simulink model "simulacao_aeropendulo_LGR"  (R2021a)
settings: Solver=ode4  StartTime=0.0  StopTime=10  FixedStep=1e-3  RelTol=1e-3
values from neighbouring files (symbols this model uses):
  b = 0.006856    [aeropendulo_vars.m]
  g = 9.81    [aeropendulo_vars.m]
  I = 0.0264    [aeropendulo_vars.m]
  kh = 2.12829e-5    (= 2.12829e-05)    [aeropendulo_vars.m]
  Lh = 0.32    [aeropendulo_vars.m]
  m = 0.3182    [aeropendulo_vars.m]
  omega_barra = sqrt(m*g*sin(theta_barra)/(kh))    [aeropendulo_vars.m]
  theta_barra = theta_deg*pi/180    (= 1.3962634016)    [aeropendulo_vars.m]
libraries: aerolibconvert2 x1
settings Model: Creator=Luis Costa  LastModifiedBy=Luis Costa

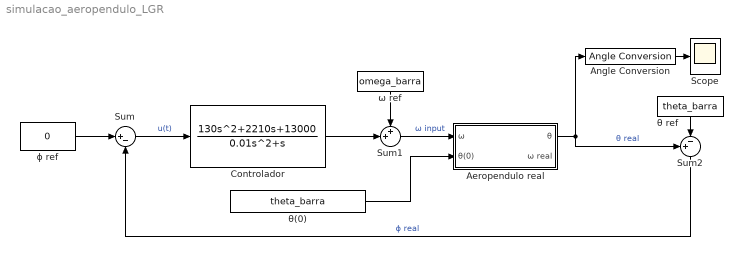
== system simulacao_aeropendulo_LGR ==
  Aeropendulo real : Subsystem
  Angle Conversion : aerolibconvert2/Angle Conversion  IU=rad  OU=deg
  Controlador : TransferFcn  Numerator=[130 2210 13000]  Denominator=[0.01 1 0]
  Scope : Scope
  Sum : Sum  Inputs=|+-
  Sum1 : Sum  Inputs=++|
  Sum2 : Sum  Inputs=+-|
  θ ref : Constant  Value=theta_barra
  θ(0) : Constant  Value=theta_barra
  ω ref : Constant  Value=omega_barra
  ϕ ref : Constant  Value=0
  wires:
  ω ref/1 -> Sum1/1
  θ ref/1 -> Sum2/2
  Sum1/1 -> Aeropendulo real/1(ω)  "ω input"
  Sum2/1 -> Sum/2  "ϕ real"
  Aeropendulo real/1(θ) -> Sum2/1, Angle Conversion/1  "θ real"
  Angle Conversion/1 -> Scope/1
  Sum/1 -> Controlador/1  "u(t)"
  θ(0)/1 -> Aeropendulo real/2(θ(0))
  ϕ ref/1 -> Sum/1
  Controlador/1 -> Sum1/2

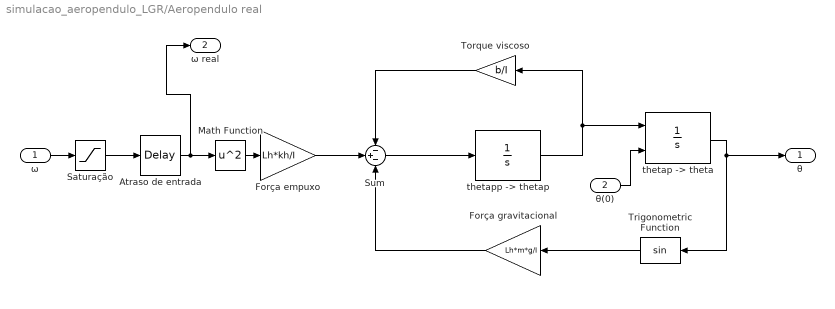
== system simulacao_aeropendulo_LGR/Aeropendulo real ==
  ω : Inport
  θ(0) : Inport  Port=2
  Atraso de entrada : TransportDelay  DelayTime=5e-3
  Força empuxo : Gain  Gain=Lh*kh/I  OutMin=[0]  OutMax=[375]
  Força gravitacional : Gain  Gain=Lh*m*g/I
  Math Function : Math  Operator=square  SaturateOnIntegerOverflow=on
  Saturação : Saturate  UpperLimit=400  LowerLimit=0
  Sum : Sum  Inputs=-+-
  Torque viscoso : Gain  Gain=b/I
  Trigonometric Function : Trigonometry
  "thetap -> theta" : Integrator  InitialConditionSource=external  UpperSaturationLimit=120*pi/180
  "thetapp -> thetap" : Integrator
  θ : Outport
  ω real : Outport  Port=2
  wires:
  "thetapp -> thetap"/1 -> Torque viscoso/1, "thetap -> theta"/1
  Força empuxo/1 -> Sum/2
  Trigonometric Function/1 -> Força gravitacional/1
  Math Function/1 -> Força empuxo/1
  Força gravitacional/1 -> Sum/3
  Torque viscoso/1 -> Sum/1
  Sum/1 -> "thetapp -> thetap"/1
  "thetap -> theta"/1 -> Trigonometric Function/1, θ/1
  ω/1 -> Saturação/1
  Saturação/1 -> Atraso de entrada/1
  Atraso de entrada/1 -> ω real/1, Math Function/1
  θ(0)/1 -> "thetap -> theta"/2
